simulink model "my747controller_discretization"  (R2021b)
settings: Solver=ode45  StartTime=0.0  StopTime=200  RelTol=1e-3
undefined symbols (not defined in the file): A, B, C, Kdisc, Ts
settings Model: Creator=tanzc  LastModifiedBy=tanzc
settings DataIOCC: LimitDataPoints=on  SaveFormat=Array  ReturnWorkspaceOutputs=off

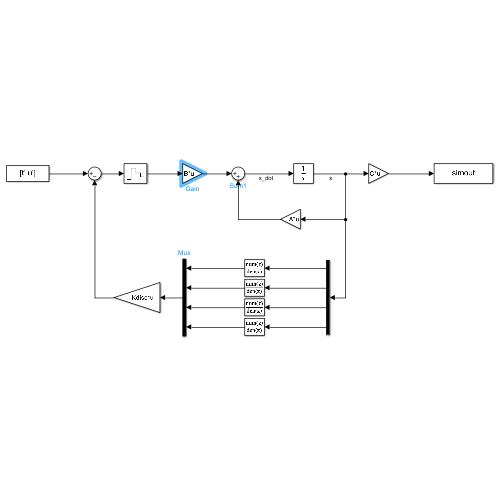
[thumbnail: Simulink's stored preview of the top-level diagram]
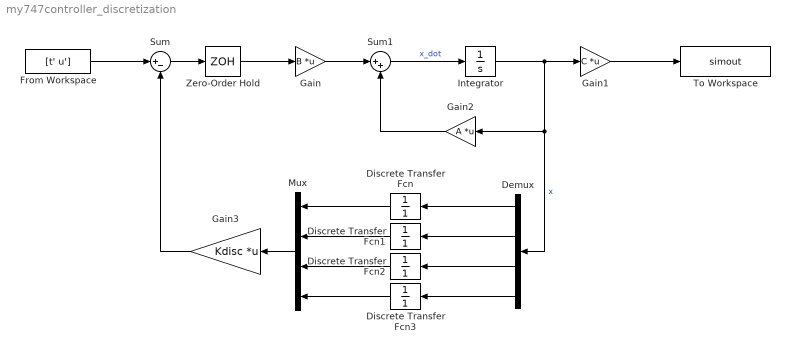
== system my747controller_discretization ==
  Demux : Demux
  Discrete Transfer Fcn{,1..3} (4 alike) : DiscreteTransferFcn  Denominator=[1]  SampleTime=Ts
  From Workspace : FromWorkspace  VariableName=[t' u']
  Gain : Gain  Gain=B  Multiplication=Matrix(K*u)
  Gain1 : Gain  Gain=C  Multiplication=Matrix(K*u)
  Gain2 : Gain  Gain=A  Multiplication=Matrix(K*u)
  Gain3 : Gain  Gain=Kdisc  Multiplication=Matrix(K*u)
  Integrator : Integrator
  Mux : Mux
  Sum : Sum  Inputs=|+-
  Sum1 : Sum  Inputs=|++
  To Workspace : ToWorkspace  VariableName=simout  SaveFormat=Structure With Time  SampleTime=-1
  Zero-Order Hold : ZeroOrderHold  SampleTime=Ts
  wires:
  Integrator/1 -> Demux/1, Gain2/1, Gain1/1  "x"
  Gain/1 -> Sum1/1
  Sum1/1 -> Integrator/1  "x_dot"
  Gain2/1 -> Sum1/2
  Gain3/1 -> Sum/2
  From Workspace/1 -> Sum/1
  Gain1/1 -> To Workspace/1
  Sum/1 -> Zero-Order Hold/1
  Zero-Order Hold/1 -> Gain/1
  Mux/1 -> Gain3/1
  Discrete Transfer Fcn/1 -> Mux/1
  Discrete Transfer Fcn1/1 -> Mux/2
  Discrete Transfer Fcn2/1 -> Mux/3
  Discrete Transfer Fcn3/1 -> Mux/4
  Demux/1 -> Discrete Transfer Fcn/1
  Demux/2 -> Discrete Transfer Fcn1/1
  Demux/3 -> Discrete Transfer Fcn2/1
  Demux/4 -> Discrete Transfer Fcn3/1
